simulink model "Model"  (R2024b)
settings: Solver=VariableStepAuto  StartTime=0.0  StopTime=10.0  RelTol=1e-3
settings Model: Creator=yugan  LastModifiedBy=sumit
settings RTWCC: GPUComputeCapability=3.5

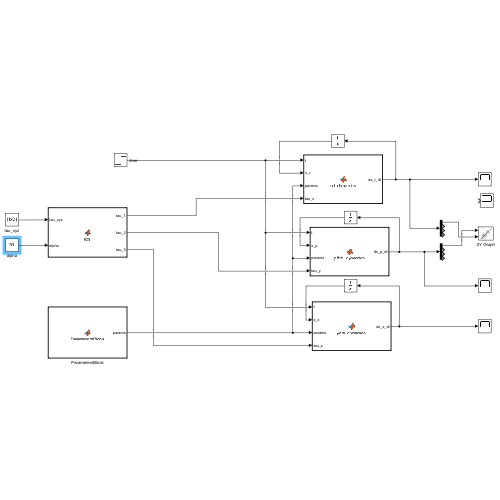
[thumbnail: Simulink's stored preview of the top-level diagram]
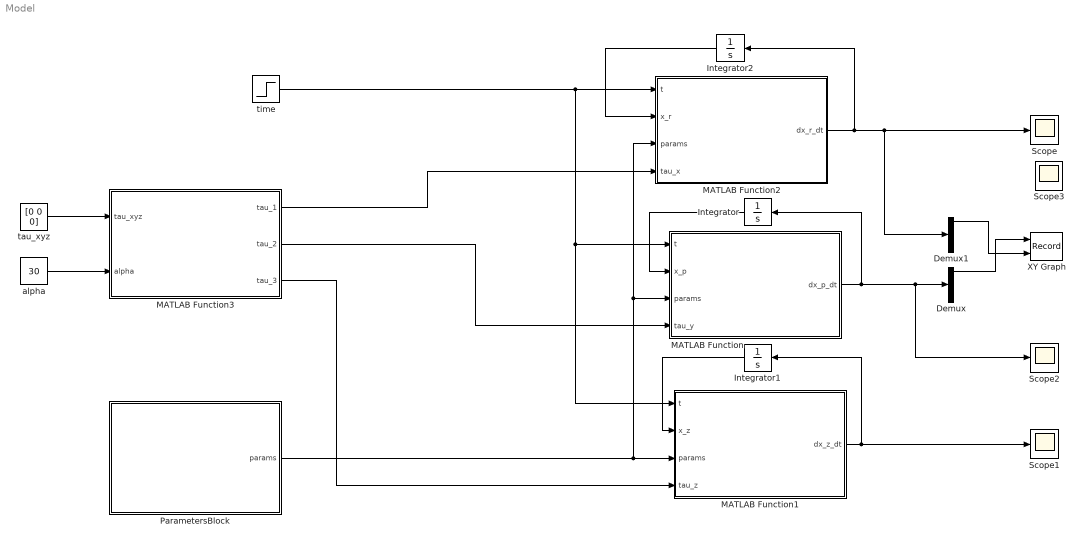
== system Model ==
  Demux : Demux
  Demux1 : Demux
  Integrator : Integrator  InitialCondition=[0; -0.1; 0; 0]
  Integrator1 : Integrator  InitialCondition=[0 ;0]
  Integrator2 : Integrator  InitialCondition=[0; 0.1; 0; 0]
  MATLAB Function : MATLAB Function  TreatAsAtomicUnit=on
  MATLAB Function1 : MATLAB Function  TreatAsAtomicUnit=on
  MATLAB Function2 : MATLAB Function  TreatAsAtomicUnit=on
  MATLAB Function3 : MATLAB Function  TreatAsAtomicUnit=on
  ParametersBlock : MATLAB Function  TreatAsAtomicUnit=on
  Scope{,1..3} (4 alike) : Scope
  XY Graph : Record  FileSettingsInternal="{\"entries\":[{\"content\":{\"excelSettings\":{\"content\":{},\"type\":\"Streamout.ExcelSettings\"}},\"type\":\"Streamout.FileSettingStorage\",\"uuid\":\"\"}],\"packageUris\":[\"http:\\/\\/schema.mathworks.com\\/mf0\\/streamout_blocks\\/R2020a\"],\"version\":\"1.0\"}"  Layout=[1 1]  SignalsInternal="{\"entries\":[{\"content\":{\"signals\":[{\"content\":{\"blockPath\":[],\"dimensions\":[1,1],\"domain\":\"\",\"lineColor\":\"#a2142f\",\"plots\":[ 1 ],\"port\":1,\"signalID\":1,\"signalName\":\"Demux:1\"},\"type\":\"RecordBlkView.Signal\",\"uuid\":\"\"},{\"content\":{\"blockPath\":[],\"dimensions\":[1,1],\"domain\":\"\",\"lineColor\":\"#139fff\",\"plots\":[ 1 ],\"port\":2,\"signalID\":2,\"signalName\":\"Demux1:1\"},\"type\":\"RecordBlkView.Signal\",\"uuid\":\"\"}]},\"type\":\"RecordBlkView.InputSignals\",\"uuid\":\"\"}],\"packageUris\":[\"http:\\/\\/schema.mathworks.com\\/mf0\\/streamout_blocks\\/R2020a\"],\"version\":\"1.0\"}"  VisualizationBindings="{\"xyplotplugin\":{\"info\":[{\"series\":[{\"bindingParametersList\":[{\"parameter\":\"X-Axis\",\"signalID\":1,\"signalName\":\"Demux:1\"},{\"parameter\":\"Y-Axis\",\"signalID\":2,\"signalName\":\"Demux1:1\"}],\"seriesID\":0}],\"subplotID\":1}]}}"  CompatibilityTag=XY
  alpha : Constant  Value=30
  tau_xyz : Constant  Value=[0 0 0]
  time : Step  After=10  SampleTime=0
  wires:
  MATLAB Function/1(dx_p_dt) -> Integrator/1, Demux/1, Scope2/1
  Integrator/1 -> MATLAB Function/2(x_p)
  MATLAB Function1/1(dx_z_dt) -> Integrator1/1, Scope1/1
  Integrator1/1 -> MATLAB Function1/2(x_z)
  MATLAB Function2/1(dx_r_dt) -> Demux1/1, Scope/1, Integrator2/1
  Integrator2/1 -> MATLAB Function2/2(x_r)
  alpha/1 -> MATLAB Function3/2(alpha)
  MATLAB Function3/1(tau_1) -> MATLAB Function2/4(tau_x)
  MATLAB Function3/2(tau_2) -> MATLAB Function/4(tau_y)
  MATLAB Function3/3(tau_3) -> MATLAB Function1/4(tau_z)
  time/1 -> MATLAB Function1/1(t), MATLAB Function/1(t), MATLAB Function2/1(t)
  ParametersBlock/1(params) -> MATLAB Function2/3(params), MATLAB Function/3(params), MATLAB Function1/3(params)
  tau_xyz/1 -> MATLAB Function3/1(tau_xyz)
  Demux/1 -> XY Graph/1
  Demux1/1 -> XY Graph/2

== matlab function Model/MATLAB Function1 ==
  data: t input; dx_z_dt output; x_z input; params input; tau_z input
function dx_z_dt = yaw_dynamics(t, x_z, params, tau_z)
% yaw_dynamics.m
%
% Implements the 1-DOF dynamic equation for the Ball Segway in the x-y
% plane (yaw motion), based on Eq. 13 (page 10).
%
% State vector x_z = [theta_z, theta_z_dot]'
% Output dx_z_dt is the derivative of the state vector.

% 1. Unpack State Vector and Parameters
theta_z     = x_z(1);
theta_z_dot = x_z(2);

% Unpack parameters from struct
I_k_param = params.I_k; I_z = params.I_z; I_w = params.I_w;
r_k = params.r_k; r_w = params.r_w; alpha_rad = params.alpha_rad;

% 2. Define Equation (from Eq. 13, page 10)
% theta_z_ddot = (I_k / (I_k*I_z + 3*(I_k+I_z)*I_w*(r_k/r_w)^2*sin(alpha)^2)) * (r_k/r_w) * tau_z

numerator = I_k_param * (r_k / r_w) * tau_z;
denominator = I_k_param * I_z + 3 * (I_k_param + I_z) * I_w * (r_k / r_w)^2 * sin(alpha_rad)^2;

theta_z_ddot = numerator / denominator;

% 3. Assemble State Derivative Vector
dx_z_dt = zeros(2, 1);
dx_z_dt(1) = theta_z_dot;
dx_z_dt(2) = theta_z_ddot;

end

== matlab function Model/MATLAB Function ==
  data: t input; dx_p_dt output; x_p input; params input; tau_y input
function dx_p_dt = pitch_dynamics(t, x_p, params, tau_y)
% pitch_dynamics.m
%
% Implements the 2-DOF dynamic equations for the Ball Segway in the x-z
% plane (pitch motion), based on Eq. 8 (page 8).
%
% State vector x_p = [x_k, theta_y, x_k_dot, theta_y_dot]'
% Output dx_p_dt is the derivative of the state vector.


% 1. Unpack State Vector and Parameters
x_k         = x_p(1);
theta_y     = x_p(2);
x_k_dot     = x_p(3);
theta_y_dot = x_p(4);
q_y_dot     = [x_k_dot; theta_y_dot];

% Unpack parameters from struct
m_a = params.m_a; m_k = params.m_k; l = params.l; I_y = params.I_y;
I_w = params.I_w; r_k = params.r_k; r_w = params.r_w;
alpha_rad = params.alpha_rad; g = params.g; I_k_param = params.I_k;

% 2. Define Matrices (from Eq. 8, page 8)

% M(q_y) - Mass Matrix
M11 = m_k + (I_k_param / r_k^2) + m_a + (3*I_w*cos(alpha_rad)^2) / (2*r_w^2);
M12 = m_a*l*cos(theta_y) - (3*I_w*cos(alpha_rad)^2) / (2*r_w^2) * r_k;
M21 = M12;
M22 = m_a*l^2 + (3*I_w*r_k^2*cos(alpha_rad)^2) / (2*r_w^2) + I_y;
M_y = [M11, M12; M21, M22];

% C(q_y, q_y_dot) - Coriolis-Centrifugal Vector
C11 = 0;
C12 = -m_a * l * theta_y_dot * sin(theta_y);
C21 = 0;
C22 = 0;
C_y = [C11, C12; C21, C22];

% G(q_y) - Gravity Vector
G1 = 0;
G2 = -m_a * g * l * sin(theta_y);
G_y = [G1; G2];

% D(q_y_dot) - Friction Vector
% Omitted as coefficients are not provided in Table 1.
D_y = [0; 0];

% Q_y - Control Torque Vector
Q1 = -(1 / r_w) * tau_y;
Q2 = (r_k / r_w) * tau_y;
Q_y = [Q1; Q2];

% 3. Calculate Accelerations
% M * q_ddot + C * q_dot + D + G = Q
% M * q_ddot = Q - C * q_dot - D - G
q_y_ddot = M_y \ (Q_y - C_y * q_y_dot - D_y - G_y); % Using \ is more stable than inv(M)

% 4. Assemble State Derivative Vector
dx_p_dt = zeros(4, 1);
dx_p_dt(1) = x_k_dot;
dx_p_dt(2) = theta_y_dot;
dx_p_dt(3) = q_y_ddot(1); % x_k_ddot
dx_p_dt(4) = q_y_ddot(2); % theta_y_ddot

end

== matlab function Model/MATLAB Function2 ==
  data: t input; dx_r_dt output; x_r input; params input; tau_x input
function dx_r_dt = roll_dynamics(t, x_r, params, tau_x)
% roll_dynamics.m
%
% Implements the 2-DOF dynamic equations for the Ball Segway in the y-z
% plane (roll motion), based on Eq. 7 (page 6).
%
% State vector x_r = [y_k, theta_x, y_k_dot, theta_x_dot]'
% Output dx_r_dt is the derivative of the state vector.


% 1. Unpack State Vector and Parameters
y_k         = x_r(1);
theta_x     = x_r(2);
y_k_dot     = x_r(3);
theta_x_dot = x_r(4);
q_x_dot     = [y_k_dot; theta_x_dot];

% Unpack parameters from struct
m_a = params.m_a; m_k = params.m_k; l = params.l; I_x = params.I_x;
I_w = params.I_w; r_k = params.r_k; r_w = params.r_w;
alpha_rad = params.alpha_rad; g = params.g; I_k_param = params.I_k;

% 2. Define Matrices (from Eq. 7, page 6)

% M(q_x) - Mass Matrix
M11 = m_k + (I_k_param / r_k^2) + m_a + (3*I_w*cos(alpha_rad)^2) / (2*r_w^2);
M12 = (3*I_w*cos(alpha_rad)^2) / (2*r_w^2) * r_k - m_a*l*cos(theta_x);
M21 = M12;
M22 = m_a*l^2 + (3*I_w*r_k^2*cos(alpha_rad)^2) / (2*r_w^2) + I_x;
M_x = [M11, M12; M21, M22];

% C(q_x, q_x_dot) - Coriolis-Centrifugal Vector
C11 = 0;
C12 = m_a * l * theta_x_dot * sin(theta_x);
C21 = 0;
C22 = 0;
C_x = [C11, C12; C21, C22];

% G(q_x) - Gravity Vector
G1 = 0;
G2 = -m_a * g * l * sin(theta_x);
G_x = [G1; G2];

% D(q_x_dot) - Friction Vector
% Omitted as coefficients are not provided in Table 1.
D_x = [0; 0];

% Q_x - Control Torque Vector
Q1 = (1 / r_w) * tau_x;
Q2 = (r_k / r_w) * tau_x;
Q_x = [Q1; Q2];

% 3. Calculate Accelerations
% M * q_ddot + C * q_dot + D + G = Q
% M * q_ddot = Q - C * q_dot - D - G
q_x_ddot = M_x \ (Q_x - C_x * q_x_dot - D_x - G_x); % Using \ is more stable than inv(M)

% 4. Assemble State Derivative Vector
dx_r_dt = zeros(4, 1);
dx_r_dt(1) = y_k_dot;
dx_r_dt(2) = theta_x_dot;
dx_r_dt(3) = q_x_ddot(1); % y_k_ddot
dx_r_dt(4) = q_x_ddot(2); % theta_x_ddot

end

== matlab function Model/MATLAB Function3 ==
  data: tau_xyz input; tau_1 output; alpha input; tau_2 output; tau_3 output
function [tau_1, tau_2, tau_3] = fcn(tau_xyz, alpha)
% --- Pre-calculate trigonometric terms ---
c_alpha = cos(alpha);
s_alpha = sin(alpha);
sqrt3 = sqrt(3);

% --- Handle potential division by zero ---
% Add a small number (epsilon) to prevent Inf if cos(a) or sin(a) is zero.
if abs(c_alpha) < eps
    c_alpha = sign(c_alpha) * eps; % Keep the sign, but use eps
    if c_alpha == 0 % Handle case where c_alpha was exactly 0
        c_alpha = eps;
    end
end
if abs(s_alpha) < eps
    s_alpha = sign(s_alpha) * eps; % Keep the sign
    if s_alpha == 0 % Handle case where s_alpha was exactly 0
        s_alpha = eps;
    end
end

% --- Define the Matrix M ---
M = [ (2 / (3 * c_alpha)) , 0                    , (1 / (3 * s_alpha));
      (-1 / (3 * c_alpha)), (sqrt3 / (3 * c_alpha)), (1 / (3 * s_alpha));
      (-1 / (3 * c_alpha)), (-sqrt3 / (3 * c_alpha)), (1 / (3 * s_alpha)) ];
      
% --- Perform the matrix multiplication ---
% Ensure tau_xyz is a column vector for correct matrix math
tau_123 = M * tau_xyz(:);

% --- Assign to separate outputs ---
tau_1 = tau_123(1);
tau_2 = tau_123(2);
tau_3 = tau_123(3);

== matlab function Model/ParametersBlock ==
  data: params output Bus: ParamsBus
function params = ParametersBlock
%#codegen

params.m_a       = 68;
params.m_k       = 19.6;
params.l         = 0.38;
params.I_x       = 12.1;
params.I_y       = 11.67;
params.I_z       = 1.08;
params.r_w       = 0.1;
params.I_w       = 0.26;
params.r_k       = 0.22;
params.I_k       = 0.38;
params.alpha     = 65.5;
params.alpha_rad = 65.5 * (pi/180);
params.g         = 9.81;
